simulink model "TVCComplete"  (R2023b)
settings: Solver=VariableStepAuto  StartTime=0.0  StopTime=10.0  RelTol=1e-3
libraries: simulink_extras x3, spsDiscreteVariableTimeDelayLib x1, slpidlib x1
settings Model: Creator=ASUS  LastModifiedBy=ASUS

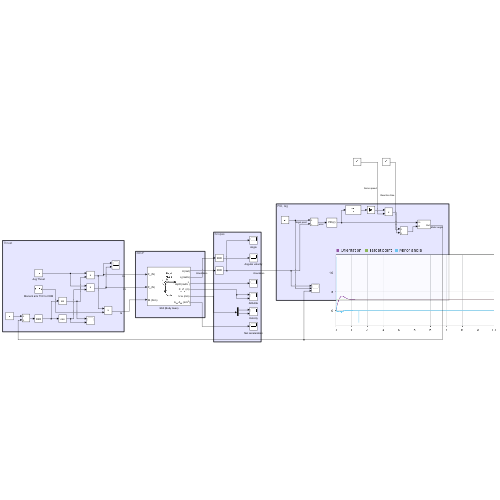
[thumbnail: Simulink's stored preview of the top-level diagram]
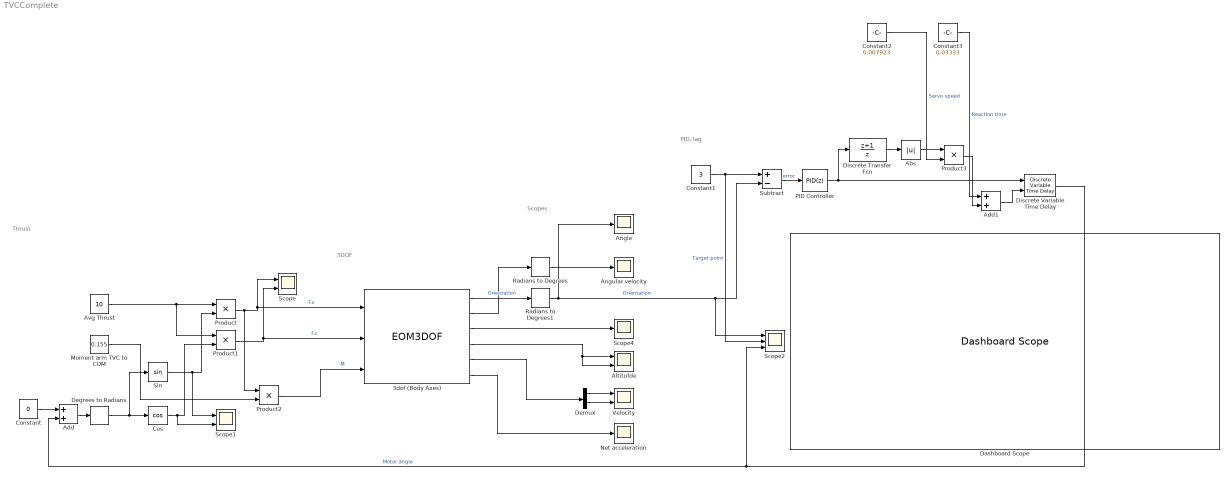
== system TVCComplete ==
  note: PID, lag
  note: Scopes
  note: 3DOF
  note: Thrust
  3dof (Body Axes) : EOM3DOF  mass=0.405  Iyy=0.006951
  Abs : Abs  SaturateOnIntegerOverflow=off
  Add : Sum
  Add1 : Sum
  Altitufde : Scope  NumInputPorts=2
  Angle : Scope
  Angular velocity : Scope
  Avg Thrust : Constant  Value=10
  Constant : Constant  Value=0
  Constant1 : Constant  Value=3
  Constant2 : Constant  Value=0.007923
  Constant3 : Constant  Value=0.03333
  Cos : Trigonometry  Operator=cos
  Dashboard Scope : DashboardScope
  Degrees to Radians : simulink_extras/Transformations/Degrees to Radians
  Demux : Demux  Outputs=2
  Discrete Transfer Fcn : DiscreteTransferFcn  Numerator=[1 1]  Denominator=[1 0]
  Discrete Variable Time Delay : spsDiscreteVariableTimeDelayLib/Discrete Variable Time Delay  MaxDelay=1  InitialValue=0  Ts=50e-6  DFT=on
      settings: LibrarySourceBlock=|
      | sps_lib/Control/Discrete Variable
      | Time Delay
  Moment arm TVC to COM : Constant  Value=0.155
  Net acceleration : Scope
  PID Controller : slpidlib/PID Controller  Controller=PID  Form=Parallel  TimeDomain=Discrete-time  UseExternalTs=off  SampleTime=-1  IntegratorMethod=Forward Euler  FilterMethod=Forward Euler  ControllerParametersSource=internal  P=0.246875  I=0.43875  UseKiTs=off  D=0.0403125  N=100  UseFilter=on  TunerSelectOption=Transfer Function Based (PID Tuner App)  InitialConditionSource=internal  InitialConditionForIntegrator=0  InitialConditionForFilter=0  DifferentiatorICPrevScaledInput=0  ExternalReset=none  TrackingMode=off  Kt=1  LimitOutput=off  SatLimitsSource=internal  UpperSaturationLimit=inf  LowerSaturationLimit=-inf  LinearizeAsGain=on  AntiWindupMode=none  Kb=1  LimitIntegrator=off  UpperIntegratorSaturationLimit=inf  LowerIntegratorSaturationLimit=-inf  POutMin=[]  POutMax=[]  IOutMin=[]  IOutMax=[]  DOutMin=[]  DOutMax=[]  NOutMin=[]  NOutMax=[]  SumOutMin=[]  SumOutMax=[]  SaturationOutMin=[]  SaturationOutMax=[]  PParamMin=[]  PParamMax=[]  IParamMin=[]  IParamMax=[]  DParamMin=[]  DParamMax=[]  NParamMin=[]  NParamMax=[]  KbParamMin=[]  KbParamMax=[]  KtParamMin=[]  KtParamMax=[]  KbOutMin=[]  KbOutMax=[]  KtOutMin=[]  KtOutMax=[]  IntegratorOutMin=[]  IntegratorOutMax=[]  FilterOutMin=[]  FilterOutMax=[]  SumI1OutMin=[]  SumI1OutMax=[]  SumI2OutMin=[]  SumI2OutMax=[]  SumI3OutMin=[]  SumI3OutMax=[]  SumI4OutMin=[]  SumI4OutMax=[]  SumDOutMin=[]  SumDOutMax=[]  DifferentiatorOutMin=[]  DifferentiatorOutMax=[]  FilterDiffOutCoefMin=[]  FilterDiffOutCoefMax=[]  ReciprocalOutMin=[]  ReciprocalOutMax=[]  SumDenOutMin=[]  SumDenOutMax=[]  SumNumOutMin=[]  SumNumOutMax=[]  DivideOutMin=[]  DivideOutMax=[]  UdiffTsProdOutMin=[]  UdiffTsProdOutMax=[]  NTsProdOutMin=[]  NTsProdOutMax=[]  UintegralTsProdOutMin=[]  UintegralTsProdOutMax=[]  UngainTsProdOutMin=[]  UngainTsProdOutMax=[]  ClampingZeroOutDataTypeStr=Inherit: Inherit via back propagation  ClampingZeroOutMin=[]  ClampingZeroOutMax=[]  FilterDenConstantOutDataTypeStr=Inherit: Inherit via back propagation  FilterDenConstantOutMin=[]  FilterDenConstantOutMax=[]  PCopyOutDataTypeStr=Inherit: Inherit via back propagation  PCopyOutMin=[]  PCopyOutMax=[]  NCopyOutDataTypeStr=Inherit: Inherit via back propagation  NCopyOutMin=[]  NCopyOutMax=[]  IntegratorContinuousStateAttributes=''  IntegratorStateMustResolveToSignalObject=off  IntegratorRTWStateStorageClass=Auto  FilterContinuousStateAttributes=''  FilterStateMustResolveToSignalObject=off  FilterRTWStateStorageClass=Auto  ParallelPVariant=InternalParameters  IdealPVariant=Disabled  IVariant=InternalParameters  DVariant=InternalParameters  IntegratorVariant=Discrete  SatVariant=Disabled  AWVariant=Passthrough  PCopyVariant=Disabled  TRVariant=Disabled  FdbkBlocksVariant=Forward  IdealPFdbkVariant=Disabled  SatFdbkVariant=Disabled  DerivativeFilterVariant=ForwardEulerFilter  NVariant=InternalParameters  NCopyVariant=Disabled  FilterICVariant=InternalICsFilter  IntegratorICVariant=InternalICs  ExternalResetVariant=Disabled  TRSumVariant=Passthrough  SumFdbkVariant=Disabled  SumVariant=Sum_PID  TsampFilterVariant=InternalTs  TsampNgainVariant=Passthrough  TsampIntegralVariant=Disabled_SignalSpec  ExternalSaturationOutDataTypeStr=Inherit: Same as second input
  Product{,1..3} (4 alike) : Product
  Radians to Degrees : simulink_extras/Transformations/Radians to Degrees
  Radians to Degrees1 : simulink_extras/Transformations/Radians to Degrees
  Scope : Scope  NumInputPorts=2
  Scope1 : Scope  NumInputPorts=2
  Scope2 : Scope  NumInputPorts=3
  Scope4 : Scope
  Sin : Trigonometry
  Subtract : Sum  Inputs=+-
  Velocity : Scope  NumInputPorts=2
  wires:
  Constant/1 -> Add/1
  Add/1 -> Degrees to Radians/1
  Degrees to Radians/1 -> Sin/1, Cos/1
  Sin/1 -> Scope1/1, Product/2
  Cos/1 -> Scope1/2, Product1/2
  Avg Thrust/1 -> Product1/1, Product/1
  Moment arm TVC to COM/1 -> Product2/2
  Product/1 -> Product2/1, Scope/1, 3dof (Body Axes)/1  "Fx"
  Product1/1 -> Scope/2, 3dof (Body Axes)/2  "Fz"
  Product2/1 -> 3dof (Body Axes)/3  "M"
  3dof (Body Axes)/1 -> Radians to Degrees1/1  "Orientation"
  Radians to Degrees1/1 -> Angle/1, Subtract/2, Scope2/1  "Orientation"
  3dof (Body Axes)/2 -> Radians to Degrees/1
  Radians to Degrees/1 -> Angular velocity/1
  3dof (Body Axes)/3 -> Scope4/1
  3dof (Body Axes)/4 -> Altitufde/2, Altitufde/1
  Demux/1 -> Velocity/1
  Demux/2 -> Velocity/2
  3dof (Body Axes)/5 -> Demux/1
  3dof (Body Axes)/6 -> Net acceleration/1
  Constant1/1 -> Scope2/2, Subtract/1  "Target point"
  Subtract/1 -> PID Controller/1  "error"
  Add1/1 -> Discrete Variable Time Delay/2
  Product3/1 -> Add1/2
  PID Controller/1 -> Discrete Variable Time Delay/1, Discrete Transfer Fcn/1
  Discrete Variable Time Delay/1 -> Scope2/3, Add/2  "Motor angle"
  Constant2/1 -> Product3/2  "Servo speed"
  Constant3/1 -> Add1/1  "Reaction time"
  Abs/1 -> Product3/1
  Discrete Transfer Fcn/1 -> Abs/1
